simulink model "FlexRulerPD"  (R2023a)
settings: Solver=ode4  StartTime=0.0  StopTime=Inf  FixedStep=0.002  RelTol=1e-3  EnableMultiTasking=on
PostLoadFcn:
  | qc_set_target_type(getConfigSet(bdroot, 'QUARC Default Target Configuration'));
values from neighbouring files (symbols this model uses):
  Kd = 1    [Init.m]
  Kep = 3    [Init.m]
  Kp = 15    [Init.m]
  Ts = 0.002    [Init.m]
  wc = 20    [Init.m]
undefined symbols (not defined in the file or in its folder): HIL
libraries: cstblocks x4, quarc_library x4, simulink x1
settings Model: SimulationMode=external  ExtModeTrigDuration=10000  Creator=MLevis  LastModifiedBy=quarc_user
settings SolverCC: AlgebraicLoopSolver=TrustRegion  PositivePriorityOrder=on  AutoInsertRateTranBlk=on
settings DataIOCC: LimitDataPoints=on  SaveFormat=Array  SignalLoggingSaveFormat=ModelDataLogs  ReturnWorkspaceOutputs=off
settings OptimizationCC: ExpressionDepthLimit=2147483647  InitFltsAndDblsToZero=on
settings DebuggingCC: SaveWithParameterizedLinksMsg=none  UnderspecifiedInitializationDetection=Classic  MergeDetectMultiDrivingBlocksExec=none  SolverPrmCheckMsg=warning  MultiTaskDSMMsg=warning  MultiTaskCondExecSysMsg=none  FcnCallInpInsideContextMsg=warning  UnconnectedInputMsg=warning  UnconnectedOutputMsg=warning  UnconnectedLineMsg=warning  StateNameClashWarn=warning  SFUnexpectedBacktrackingDiag=warning  SFNoUnconditionalDefaultTransitionDiag=warning  SFExecutionAtInitializationDiag=none  ArithmeticOperatorsInVariantConditions=warning
settings ModelReferenceCC: EnableRefExpFcnMdlSchedulingChecks=on  PropagateSignalLabelsOutOfModel=off
settings SFSimCC: SimUseLocalCustomCode=off  CustomCodeUndefinedFunction=UseInterfaceOnly
settings RTWCC: Description=QUARC Win64 Target Using Toolchain  SystemTargetFile=quarc_win64.tlc  TemplateMakefile=quarc_default_tmf  RTWUseLocalCustomCode=off  Toolchain=QUARC win64 | nmake (64-bit Windows)  BuildConfiguration=Faster Runs  DLArmComputeVersion=19.05
settings CodeAppCC: StateflowObjectComments=on
settings STFCustomTargetCC: TargetLangStandard=C89/C90 (ANSI)  SystemTargetFile=quarc_win64.tlc
settings GRTTargetCC: TargetLangStandard=C89/C90 (ANSI)  ParMdlRefBuildCompliant=off  CompOptLevelCompliant=off  CombineOutputUpdateFcns=off  MatFileLogging=off  CPPClassGenCompliant=off  GRTInterface=on  ExtMode=on  ExtModeMexFile=quarc_comm
settings ConfigComp: CovMetricSettings=dw  CovSaveCumulativeToWorkspaceVar=on  CovSaveSingleToWorkspaceVar=on  CovExternalEMLEnable=off

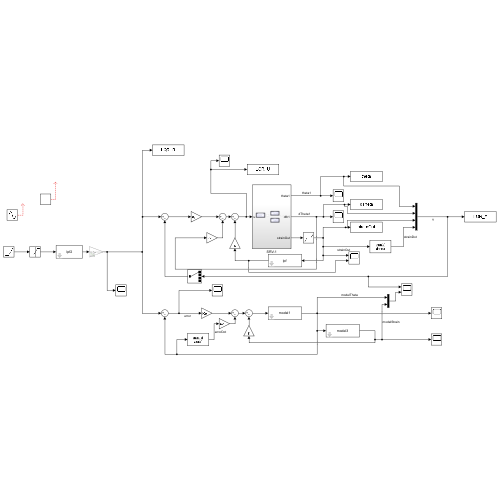
[thumbnail: Simulink's stored preview of the top-level diagram]
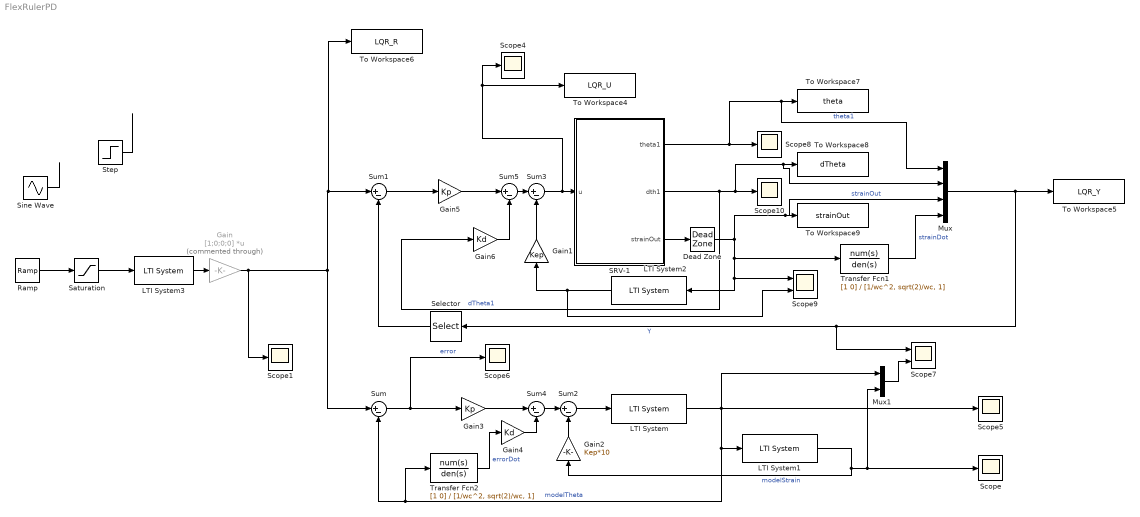
== system FlexRulerPD ==
  Dead Zone : DeadZone  LowerValue=0.05  UpperValue=0.09
  Gain : Gain  Commented=through  Gain=[1;0;0;0]  Multiplication=Matrix(K*u)
  Gain1 : Gain  Gain=Kep
  Gain2 : Gain  Gain=Kep*10
  Gain3 : Gain  Gain=Kp
  Gain4 : Gain  Gain=Kd
  Gain5 : Gain  Gain=Kp
  Gain6 : Gain  Gain=Kd
  LTI System : cstblocks/LTI System  sys=model1  IC=[]
  LTI System1 : cstblocks/LTI System  sys=model3  IC=[]
  LTI System2 : cstblocks/LTI System  sys=lpf  IC=[]
  LTI System3 : cstblocks/LTI System  sys=lpf2  IC=[]
  Mux : Mux
  Mux1 : Mux  Inputs=2
  Ramp : simulink/Sources/Ramp  slope=3.5  start=0  InitialOutput=0
  SRV-1 : Subsystem
  Saturation : Saturate  UpperLimit=1
  Scope{,1,4..6,8,10} (7 alike) : Scope
  Scope7 : Scope  NumInputPorts=2
  Scope9 : Scope  NumInputPorts=2
  Selector : Selector  InputPortWidth=4  IndexOptions=Index vector (dialog)  Indices=[1]  OutputSizes=1
  Sine Wave : Sin  Frequency=2  SampleTime=0
  Step : Step  After=0  SampleTime=0
  Sum{,1..5} (6 alike) : Sum  Inputs=|+-
  To Workspace4 : ToWorkspace  VariableName=LQR_U  SampleTime=Ts
      settings: MaxDataPoints=Te/Ts
  To Workspace5 : ToWorkspace  VariableName=LQR_Y  SampleTime=Ts
      settings: MaxDataPoints=Te/Ts
  To Workspace6 : ToWorkspace  VariableName=LQR_R  SaveFormat=Timeseries  SampleTime=-1
  To Workspace7 : ToWorkspace  VariableName=theta  SampleTime=Ts
      settings: MaxDataPoints=Te/Ts
  To Workspace8 : ToWorkspace  VariableName=dTheta  SampleTime=Ts
      settings: MaxDataPoints=Te/Ts
  To Workspace9 : ToWorkspace  VariableName=strainOut  SampleTime=Ts
      settings: MaxDataPoints=Te/Ts
  Transfer Fcn1 : TransferFcn  Numerator=[1 0]  Denominator=[1/wc^2, sqrt(2)/wc, 1]  ParameterTunability=Unconstrained
  Transfer Fcn2 : TransferFcn  Numerator=[1 0]  Denominator=[1/wc^2, sqrt(2)/wc, 1]  ParameterTunability=Unconstrained
  wires:
  Step/1 -> ?
  LTI System/1 -> Mux1/1, LTI System1/1, Transfer Fcn2/1, Sum/2, Scope5/1  "modelTheta"
  Sum/1 -> Gain3/1, Scope6/1  "error"
  Mux/1 -> Scope7/1, Selector/1, To Workspace5/1  "Y"
  Sine Wave/1 -> ?
  SRV-1/2(dth1) -> Gain6/1, Mux/2, To Workspace8/1, Scope10/1  "dTheta1"
  SRV-1/3(strainOut) -> Dead Zone/1
  SRV-1/1(theta1) -> Mux/1, To Workspace7/1, Scope8/1  "theta1"
  Transfer Fcn1/1 -> Mux/4  "strainDot"
  Gain/1 -> Scope1/1, Sum1/1, To Workspace6/1, Sum/1
  Sum1/1 -> Gain5/1
  Selector/1 -> Sum1/2
  LTI System1/1 -> Gain2/1, Mux1/2, Scope/1  "modelStrain"
  Gain2/1 -> Sum2/2
  Sum2/1 -> LTI System/1
  Sum3/1 -> To Workspace4/1, Scope4/1, SRV-1/1(u)
  Mux1/1 -> Scope7/2
  LTI System2/1 -> Scope9/2, Gain1/1
  Gain1/1 -> Sum3/2
  Transfer Fcn2/1 -> Gain4/1  "errorDot"
  Sum4/1 -> Sum2/1
  Gain3/1 -> Sum4/1
  Gain4/1 -> Sum4/2
  Gain5/1 -> Sum5/1
  Sum5/1 -> Sum3/1
  Gain6/1 -> Sum5/2
  Dead Zone/1 -> Scope9/1, LTI System2/1, Transfer Fcn1/1, Mux/3, To Workspace9/1  "strainOut"
  Ramp/1 -> Saturation/1
  LTI System3/1 -> Gain/1
  Saturation/1 -> LTI System3/1

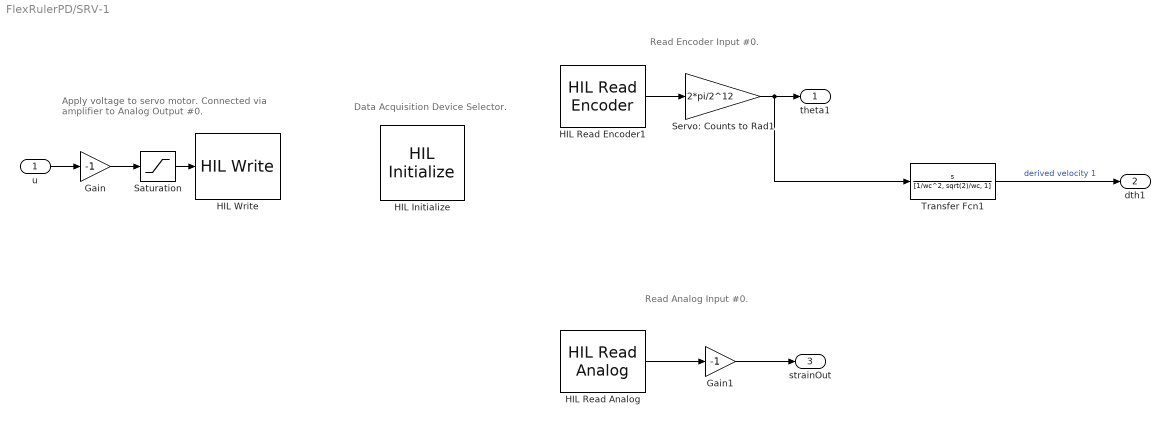
== system FlexRulerPD/SRV-1 ==
  note: Apply voltage to servo motor.
      | Connected via amplifier to Analog Output #0.
  note: Read Analog Input #0.
  note: Data Acquisition Device Selector.
  note: Read Encoder Input #0.
  u : Inport
  Gain : Gain  Gain=-1
  Gain1 : Gain  Gain=-1
  HIL Initialize : quarc_library/Data Acquisition/Generic/Configuration/HIL Initialize  object_name=HIL-1  board_type=q2_usb  board_number=0  board_options=d0=digital;d1=digital;led=auto;update_rate=normal;decimation=1  exclusive=off  active=off  hardware_clocks=[0]  clock_modes=[]  initial_clock_frequencies=[]  set_clock_params_at_start=off  set_clock_params_at_switch_in=off  set_clock_frequencies_at_start=off  set_clock_frequencies_at_switch_in=off  analog_input_channels=[0:1]  analog_input_configurations=[]  analog_input_maximums=10  analog_input_minimums=-10  set_analog_input_params_at_start=on  set_analog_input_params_at_switch_in=off  analog_output_channels=[0:1]  analog_output_maximums=10  analog_output_minimums=-10  initial_analog_outputs=[0]  final_analog_outputs=[0]  watchdog_analog_outputs=0  set_analog_output_params_at_start=on  set_analog_output_params_at_switch_in=off  set_analog_outputs_at_start=on  set_analog_outputs_at_switch_in=off  set_analog_outputs_at_terminate=on  set_analog_outputs_at_switch_out=off  set_analog_outputs_on_watchdog=off  digital_input_channels=[]  digital_output_channels=[]  digital_output_configuration=[]  initial_digital_outputs=[1]  final_digital_outputs=[1]  watchdog_digital_outputs=[1]  set_digital_output_params_at_start=off  set_digital_output_params_at_switch_in=off  set_digital_outputs_at_start=on  set_digital_outputs_at_switch_in=off  set_digital_outputs_at_terminate=on  set_digital_outputs_at_switch_out=off  set_digital_outputs_on_watchdog=off  encoder_channels=[0:1]  quadrature=[4]  encoder_filter_frequency=[]  initial_encoder_counts=[0]  set_encoder_params_at_start=on  set_encoder_params_at_switch_in=off  set_encoder_counts_at_start=on  set_encoder_counts_at_switch_in=off  pwm_channels=[]  pwm_modes=[0]  pwm_frequency=1/0.020  pwm_configuration=[]  pwm_alignment=[]  pwm_polarity=[]  pwm_leading_deadband=[]  pwm_trailing_deadband=[]  initial_pwm_outputs=[0]  final_pwm_outputs=[0]  watchdog_pwm_outputs=[0]  set_pwm_params_at_start=on  set_pwm_params_at_switch_in=off  set_pwm_outputs_at_start=on  set_pwm_outputs_at_switch_in=off  set_pwm_outputs_at_terminate=on  set_pwm_outputs_at_switch_out=off  set_pwm_outputs_on_watchdog=off  other_output_channels=[]  initial_other_outputs=[]  final_other_outputs=[]  watchdog_other_outputs=[]  set_other_outputs_at_start=off  set_other_outputs_at_switch_in=off  set_other_outputs_at_terminate=off  set_other_outputs_at_switch_out=off  set_other_outputs_on_watchdog=off
  HIL Read Analog : quarc_library/Data Acquisition/Generic/Immediate I//O/HIL Read Analog  object_name=HIL-1  channels=[0]  sample_time=qc_get_step_size  active=on  vector_output=off
  HIL Read Encoder1 : quarc_library/Data Acquisition/Generic/Immediate I//O/HIL Read Encoder  object_name=HIL-1  channels=0  sample_time=qc_get_step_size  active=on  vector_output=off  data_type_mode=Inherit via back propagation  data_type=double
  HIL Write : quarc_library/Data Acquisition/Generic/Immediate I//O/HIL Write  Tag=unassigned  object_name=HIL-1  analog_channels=0  pwm_channels=[]  digital_channels=[]  other_channels=[]  sample_time=-1  active=off  vector_input=off
  Saturation : Saturate  UpperLimit=10  LowerLimit=-10
  Servo: Counts to Rad1 : Gain  Gain=2*pi/2^12
  Transfer Fcn1 : TransferFcn  Numerator=[1 0]  Denominator=[1/wc^2, sqrt(2)/wc, 1]  ParameterTunability=Unconstrained
  theta1 : Outport
  dth1 : Outport  Port=2
  strainOut : Outport  Port=3
  wires:
  HIL Read Analog/1 -> Gain1/1
  u/1 -> Gain/1
  Saturation/1 -> HIL Write/1
  Gain/1 -> Saturation/1
  Gain1/1 -> strainOut/1
  Servo: Counts to Rad1/1 -> Transfer Fcn1/1, theta1/1
  HIL Read Encoder1/1 -> Servo: Counts to Rad1/1
  Transfer Fcn1/1 -> dth1/1  "derived velocity 1"
